simulink model "full_sensor"  (R2023b)
settings: Solver=VariableStepAuto  StartTime=0.0  StopTime=tf  RelTol=1e-3
libraries: dyn_lib x3, aerolibutil x2
settings Model: Creator=brent  LastModifiedBy=brent

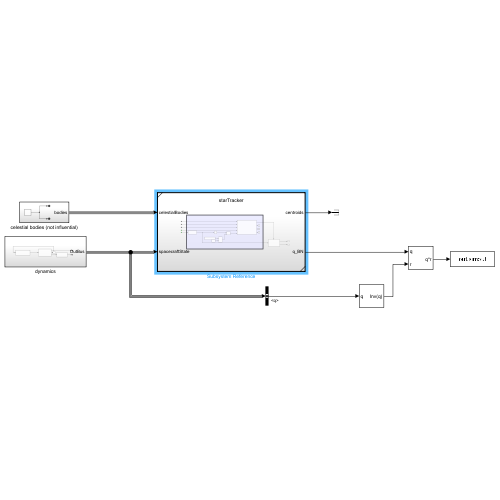
[thumbnail: Simulink's stored preview of the top-level diagram]
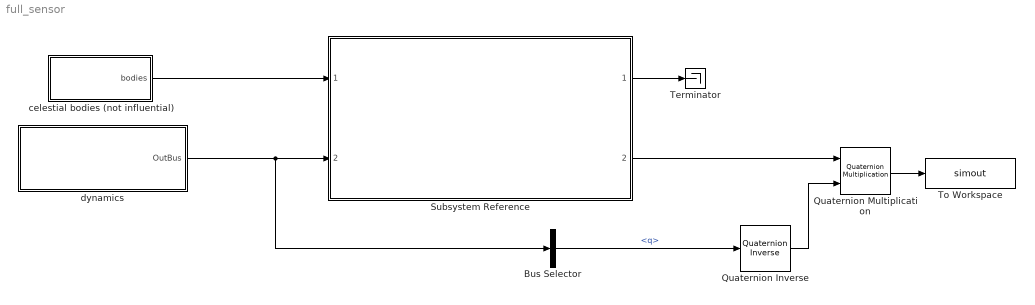
== system full_sensor ==
  Bus Selector : BusSelector  OutputSignals=q
  Quaternion Inverse : aerolibutil/Quaternion Inverse
  Quaternion Multiplication : aerolibutil/Quaternion Multiplication
  Subsystem Reference : Subsystem  TreatAsAtomicUnit=on  SystemSampleTime=1  ReferencedSubsystem=starTracker
      settings: PermitHierarchicalResolution=None
  Terminator : Terminator
  To Workspace : ToWorkspace  VariableName=simout  SaveFormat=Timeseries  SampleTime=-1
  celestial bodies (not influential) : Subsystem
  dynamics : Subsystem
  wires:
  Subsystem Reference/1 -> Terminator/1
  dynamics/1(OutBus) -> Bus Selector/1, Subsystem Reference/2
  celestial bodies (not influential)/1(bodies) -> Subsystem Reference/1
  Subsystem Reference/2 -> Quaternion Multiplication/1
  Bus Selector/1 -> Quaternion Inverse/1  "<q>"
  Quaternion Inverse/1 -> Quaternion Multiplication/2
  Quaternion Multiplication/1 -> To Workspace/1

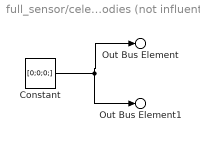
== system full_sensor/celestial bodies (not influential) ==
  Constant : Constant  Value=[0;0;0;]
  Out Bus Element : Outport  PortName=bodies  Element=Sun
  Out Bus Element1 : Outport  PortName=bodies  Element=Earth
  wires:
  Constant/1 -> Out Bus Element/1, Out Bus Element1/1

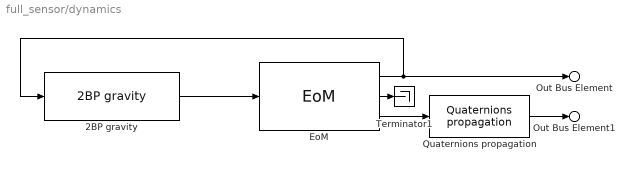
== system full_sensor/dynamics ==
  2BP gravity : dyn_lib/2BP gravity  mu=Environment.Earth.mu.value
      settings: SourceProductName=Dynamics library
  EoM : dyn_lib/EoM  x0=x0  v0=v0
      settings: SourceProductName=Dynamics library
  Quaternions propagation : dyn_lib/Quaternions propagation  q0=q0
      settings: SourceProductName=Dynamics library
  Terminator1 : Terminator
  Out Bus Element : Outport  PortName=OutBus  Element=x
  Out Bus Element1 : Outport  PortName=OutBus  Element=q
  wires:
  EoM/2 -> Terminator1/1
  EoM/3 -> Quaternions propagation/1
  EoM/1 -> Out Bus Element/1, 2BP gravity/1
  2BP gravity/1 -> EoM/1
  Quaternions propagation/1 -> Out Bus Element1/1
